simulink library "state_bus"  (R2018b)
settings: Solver=VariableStepAuto  StartTime=0.0  StopTime=10.0  RelTol=1e-3
undefined symbols (not defined in the file): q_eci2body, r_eci_km, v_eci_kmps, w_body_radps
settings Model: Creator=satcave1  LastModifiedBy=Taylor

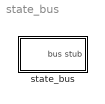
== system state_bus ==
  state_bus : Subsystem

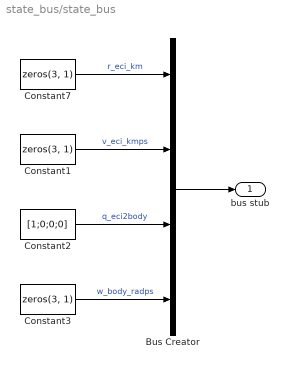
== system state_bus/state_bus ==
  Bus Creator : BusCreator  Inputs=r_eci_km,v_eci_kmps,q_eci2body,w_body_radps  OutDataTypeStr=Bus: state
  Constant1 : Constant  Value=zeros(3, 1)
  Constant2 : Constant  Value=[1;0;0;0]
  Constant3 : Constant  Value=zeros(3, 1)
  Constant7 : Constant  Value=zeros(3, 1)
  bus stub : Outport  OutDataTypeStr=Bus: state
  wires:
  Constant7/1 -> Bus Creator/1  "r_eci_km"
  Bus Creator/1 -> bus stub/1
  Constant3/1 -> Bus Creator/4  "w_body_radps"
  Constant1/1 -> Bus Creator/2  "v_eci_kmps"
  Constant2/1 -> Bus Creator/3  "q_eci2body"
